simulink model "trial_1"  (R2024b)
settings: Solver=VariableStepAuto  StartTime=0.0  StopTime=10.0  RelTol=1e-3
InitFcn:
  | run param_file.m
settings Model: Creator=user  LastModifiedBy=user

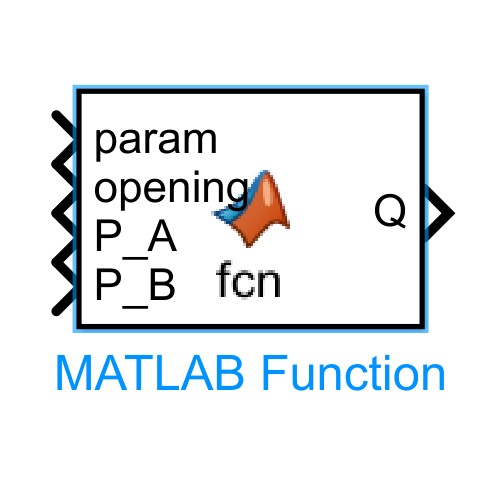
[thumbnail: Simulink's stored preview of the top-level diagram]
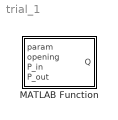
== system trial_1 ==
  MATLAB Function : MATLAB Function  TreatAsAtomicUnit=on

== matlab function trial_1/MATLAB Function ==
  data: param input; Q output; opening input; P_in input; P_out input
function Q = fcn(param, opening, P_in, P_out)

Q = param.Cd*param.Av_max*opening*sqrt(2/param.rho)*sqrt(abs(P_in-P_out))
